simulink model "G7_Reaching"  (R2023b)
settings: Solver=FixedStepDiscrete  StartTime=0.0  StopTime=inf  FixedStep=0.001  RelTol=1e-3
libraries: PhanTorque_3Dof_Library_64Bits x1, vrlib x1
settings Model: Creator=carlos.aldana  LastModifiedBy=karim
settings SolverCC: AlgebraicLoopSolver=TrustRegion
settings DataIOCC: LimitDataPoints=on  SaveFormat=Array  ReturnWorkspaceOutputs=off
settings OptimizationCC: BlockReduction=off  BooleanDataType=off  LifeSpan=inf
settings DebuggingCC: SaveWithParameterizedLinksMsg=none  UnderspecifiedInitializationDetection=Classic  MergeDetectMultiDrivingBlocksExec=none  SignalResolutionControl=TryResolveAllWithWarning  UnconnectedInputMsg=warning  UnconnectedOutputMsg=warning  UnconnectedLineMsg=warning  AllowSymbolicDim=off  SFUnexpectedBacktrackingDiag=warning  SFNoUnconditionalDefaultTransitionDiag=warning  SFExecutionAtInitializationDiag=none  ArithmeticOperatorsInVariantConditions=warning
settings HardwareCC: ProdBitPerPointer=32  ProdBitPerSizeT=32  ProdBitPerPtrDiffT=32  ProdLargestAtomicFloat=None  ProdIntDivRoundTo=Undefined  ProdEndianess=Unspecified  ProdWordSize=32  ProdHWDeviceType=32-bit Generic  TargetUnknown=on
settings ModelReferenceCC: EnableRefExpFcnMdlSchedulingChecks=on  PropagateSignalLabelsOutOfModel=off
settings SFSimCC: SimUseLocalCustomCode=off  CustomCodeUndefinedFunction=UseInterfaceOnly
settings RTWCC: RTWUseLocalCustomCode=off  DLArmComputeVersion=19.05
settings CodeAppCC: StateflowObjectComments=on
settings GRTTargetCC: TargetLangStandard=C89/C90 (ANSI)
settings ConfigComp: CovMetricSettings=dw  CovSaveCumulativeToWorkspaceVar=on  CovSaveSingleToWorkspaceVar=on  CovExternalEMLEnable=off  CovSFcnEnable=off

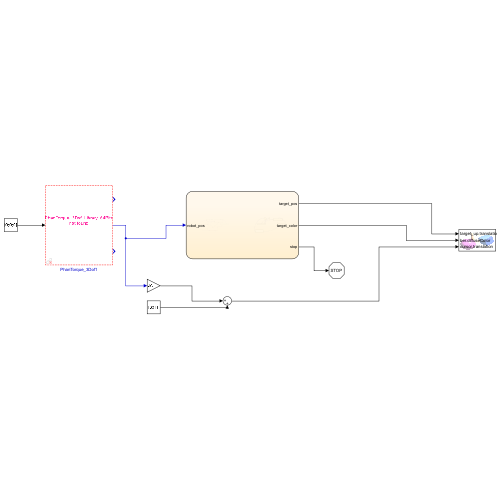
[thumbnail: Simulink's stored preview of the top-level diagram]
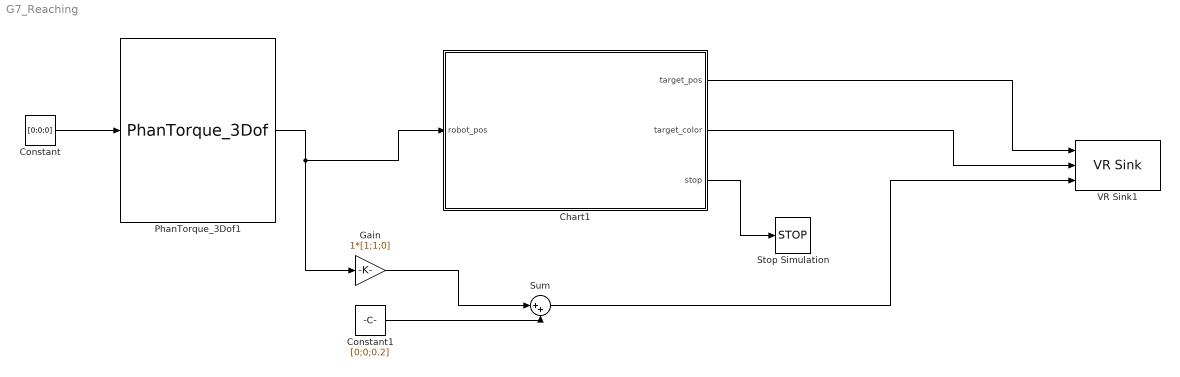
== system G7_Reaching ==
  Chart1 : Stateflow chart  TreatAsAtomicUnit=on
  Constant : Constant  Value=[0;0;0]
  Constant1 : Constant  Value=[0;0;0.2]
  Gain : Gain  Gain=1*[1;1;0]
  PhanTorque_3Dof1 : PhanTorque_3Dof_Library_64Bits/PhanTorque_3Dof  Haptic_Name='Dumbi'
  Stop Simulation : Stop
  Sum : Sum  Inputs=|++
  VR Sink1 : vrlib/VR Sink  InstantiateOnLoad=on  SampleTime=0.1  ViewEnable=on  RemoteChange=off  RemoteView=off  FieldsWritten=target_up.translation.3.1.1.double#ber.diffuseColor.3.1.1.double#cursor.translation.3.1.1.double  WorldFileName=G78_palline_color.wrl  AutoView=off  VideoDimensions=[]  AllowVariableSize=off  FigureProperties=[]
  wires:
  Chart1/1(target_pos) -> VR Sink1/1
  Chart1/2(target_color) -> VR Sink1/2
  Gain/1 -> Sum/1
  Constant1/1 -> Sum/2
  Sum/1 -> VR Sink1/3
  PhanTorque_3Dof1/2 -> Chart1/1(robot_pos), Gain/1
  Constant/1 -> PhanTorque_3Dof1/1
  Chart1/3(stop) -> Stop Simulation/1

== stateflow chart G7_Reaching/Chart1 ==
  state Start1
    entry:
    radius = 0.1;
    threshold = 0.01;
    target_color = [0 0 1];
    i = i+1;
    target_pos = [0; 0; 0];
  state Finish1
    entry:
    stop=1;
  state Hometarget2
    target_pos = [0; 0; 0];
    target_color = [0 0 1];
    distance_diff =  (robot_pos(1,1)-target_pos(1,1))^2 +(robot_pos(2,1)-target_pos(2,1))^2;
    distance = sqrt(distance_diff)
    %during:
    %distance_diff =  (robot_pos(1,1)-target_pos(1,1))^2 +(robot_pos(2,1)-target_pos(2,1))^2
    %distance = sqrt(distance_diff);
  state Start [commented out]
    entry:
    radius = 0.1;
    threshold = 0.2;
    target_color = [0 0 1];
    i = 1;
    target_pos = [0; 0; 0];
  state Finish [commented out]
  state Target [commented out]
    entry:
    target_color = [1 1 1];
    target_pos = [radius*cos(angle); radius*sin(angle); 0];
    distance_diff = (robot_pos(1,1)-target_pos(1,1))^2 +(robot_pos(2,1)-target_pos(2,1))^2;
    distance = sqrt(distance_diff);
    during:
    distance_diff = (robot_pos(1,1)-target_pos(1,1))^2 +(robot_pos(2,1)-target_pos(2,1))^2;
    distance = sqrt(distance_diff)
  state Colour_change_two1
    entry:
    target_color = [1 0 0];
    during:
    distance_diff = (robot_pos(1,1)-target_pos(1,1))^2 +(robot_pos(2,1)-target_pos(2,1))^2;
    distance = sqrt(distance_diff);
  state Colour_2
    target_color = [1 0 1];
    during:
    distance_diff = (robot_pos(1,1)-target_pos(1,1))^2 +(robot_pos(2,1)-target_pos(2,1))^2;
    distance = sqrt(distance_diff);
  state Colour_change_two [commented out]
    entry:
    target_color = [1 0 0];
    during:
    distance_diff = (robot_pos(1,1)-target_pos(1,1))^2 +(robot_pos(2,1)-target_pos(2,1))^2;
    distance = sqrt(distance_diff);
  state Colour_1 [commented out]
    target_color = [1 0 1];
    during:
    distance_diff = (robot_pos(1,1)-target_pos(1,1))^2 +(robot_pos(2,1)-target_pos(2,1))^2;
    distance = sqrt(distance_diff);
  state Hometarget [commented out]
    target_pos = [0; 0; 0];
    target_color = [0 0 1];
    distance_diff =  (robot_pos(1,1)-target_pos(1,1))^2 +(robot_pos(2,1)-target_pos(2,1))^2;
    distance = sqrt(distance_diff)
    %during:
    %distance_diff =  (robot_pos(1,1)-target_pos(1,1))^2 +(robot_pos(2,1)-target_pos(2,1))^2
    %distance = sqrt(distance_diff);
  state Target2
    entry:
    target_color = [1 1 1];
    imax = 8;
    random=randi(imax);
    angle = 2*pi/8*random;
    target_pos = [radius*cos(angle); radius*sin(angle); 0];
    distance_diff = (robot_pos(1,1)-target_pos(1,1))^2 +(robot_pos(2,1)-target_pos(2,1))^2;
    distance = sqrt(distance_diff);
    during:
    distance_diff = (robot_pos(1,1)-target_pos(1,1))^2 +(robot_pos(2,1)-target_pos(2,1))^2;
    distance = sqrt(distance_diff)
  Colour_change_two1 -> Hometarget2 : [after(1,sec) && distance<threshold]{angle = 2*pi*rand;}
  Start1 -> Target2 [order 1] : [i <20]
  Start1 -> Finish1 [order 2] : [i>=20]
  (default) -> Start1
  Start -> Finish [commented out] : [i >= 10]
  Colour_change_two -> Target [commented out] : [after(1,sec) && distance<threshold]{angle = 2*pi*rand;}
  Colour_2 -> Hometarget2 [order 2] : [distance>threshold]
  Colour_2 -> Start1 [order 1] : [after(2,sec) && distance<threshold]{i = i + 1;}
  Hometarget2 -> Colour_2 : [distance<threshold]
  Start -> Hometarget [commented out] : [i <10]
  (default) -> Start [commented out]
  Colour_1 -> Target [commented out] : [distance>threshold]
  Target -> Colour_1 [commented out] : [distance<threshold]
  Hometarget -> Target [commented out] : [distance<threshold]
  Target2 -> Colour_change_two1 : [distance<threshold]
  Colour_1 -> Hometarget [commented out] : [after(1,sec) && distance<threshold]{i = i + 1;}
  Colour_change_two -> Hometarget [commented out] : [distance>threshold]
  Hometarget -> Hometarget [commented out] : [distance>=threshold]
  data: target_pos output; target_color output; robot_pos input; angle local; distance local; i local =0; distance_diff local; threshold local double; radius local; imax local; random local; stop output
